simulink model "ActiveLoad_test"  (R2013a)
settings: Solver=ode4  StartTime=0.0  StopTime=10  FixedStep=Ts  RelTol=1e-3
PostLoadFcn:
  | Ts=100e-6; cb_mech_delay=5/60;
InitFcn:
  | Ts=100e-6; cb_mech_delay=5/60;
libraries: breaker_lib x2, powerlib x2, cables_lib x1, transformer_lib x1, alpha_betaActiveLoad_lib x1
settings Model: Creator=ch24070  LastModifiedBy=ed12083

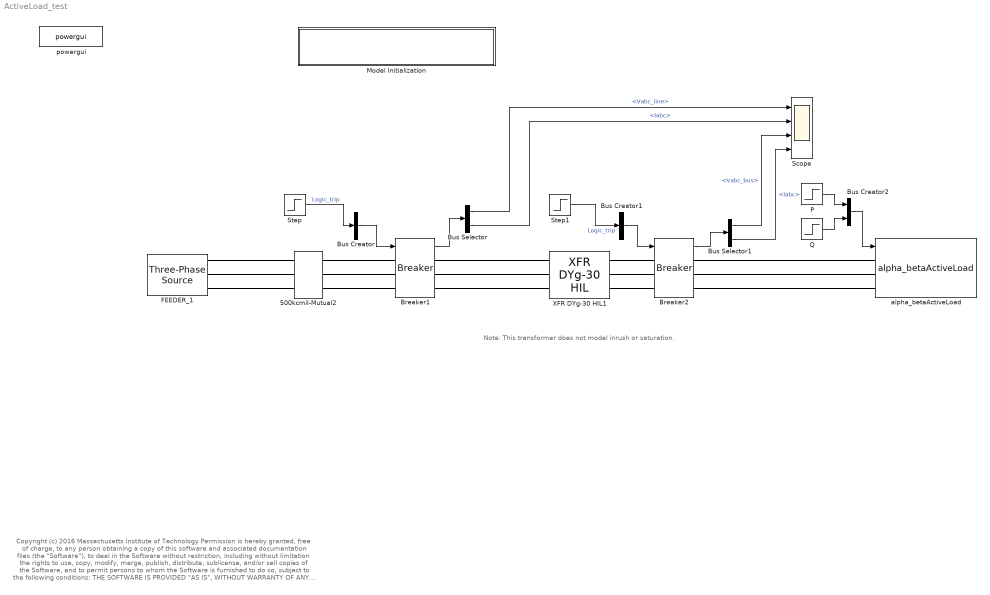
== system ActiveLoad_test ==
  note: Note: This transformer does not model inrush or saturation.
  note: Copyright (c) 2016 Massachusetts Institute of Technology
      | Permission is hereby granted, free of charge, to any person obtaining a copy of this software and associated documentation files (the "Software"), to deal
      | in the Software without restriction, including without limitation the rights to use, copy, modify, merge, publish, distribute, sublicense, and/or sell copies of the
      | Software, and to permit persons to whom the Software is furnished to do so, subject to the following conditions:
      |
      | THE SOFTWARE IS PROVIDED "AS IS", WITHOUT WARRANTY OF ANY KIND, EXPRESS OR IMPLIED, INCLUDING BUT NOT LIMITED TO THE
      | WARRANTIES OF MERCHANTABILITY, FITNESS FOR A PARTICULAR PURPOSE AND NONINFRINGEMENT. IN NO EVENT SHALL THE AUTHORS
      | OR COPYRIGHT HOLDERS BE LIABLE FOR ANY CLAIM, DAMAGES OR OTHER LIABILITY, WHETHER IN AN ACTION OF CONTRACT, TORT OR
      | OTHERWISE, ARISING FROM, OUT OF OR IN CONNECTION WITH THE SOFTWARE OR THE USE OR OTHER DEALINGS IN THE SOFTWARE.
  500kcmil-Mutual2 : cables_lib/500kcmil-Mutual  length=5000  par_sets=1  ratio=3
  Breaker1 : breaker_lib/Breaker  Ts=Ts  mech_delay=cb_mech_delay
  Breaker2 : breaker_lib/Breaker  Ts=Ts  mech_delay=cb_mech_delay
  Bus Creator : BusCreator  Inputs=1
  Bus Creator1 : BusCreator  Inputs=1
  Bus Creator2 : BusCreator  Inputs=2
  Bus Selector : BusSelector  OutputSignals=Vabc_line,Iabc
  Bus Selector1 : BusSelector  OutputSignals=Vabc_bus,Iabc
  FEEDER_1 : powerlib/Electrical Sources/Three-Phase Source  Voltage=13800  PhaseAngle=0  Frequency=60  InternalConnection=Yg  SpecifyImpedance=on  Resistance=0.8929  Inductance=16.58e-3  ShortCircuitLevel=375e6  BaseVoltage=13800  XRratio=7.9  BusType=swing  Pref=0  Qref=0  Qmin=-inf  Qmax=inf
  Model Initialization : Subsystem  AncestorBlock=artemis/Tools /Misc/Model Initialization  mask(Model Functions){InitFcnX=Ts=100e-6; cb_mech_delay=5/60;, prel=off, posl=on, inif=on, strf=off}
      mask prompts: InitFcnX "Initialisation"; prel "Preload Function"; posl "PostLoad Function"; inif "InitFcn"; strf "StartFcn"
      mask init:
      | currentBlock = gcb;
      | root = bdroot(currentBlock);
      | 
      | 
      | if ~strcmp(get_param(root,'BlockDiagramType'),'library')
      |     if prel==1
      |         set_param(root, 'PreLoadFcn', InitFcnX);
      |     else
      |         set_param(root, 'PreLoadFcn', '');
      |     end
      |     if inif==1
      |         set_param(root, 'InitFcn', InitFcnX);
      |     else
      |         set_param(root, 'InitFcn', '');
      |     end
      |     if strf==1
      |         set_param(root, 'StartFcn', InitFcnX);
      |     else
      |         set_param(root, 'StartFcn', '');
      |     end
      |     if posl==1
      |         set_param(root, 'PostLoadFcn', InitFcnX);
      |     else
      |         set_param(root, 'PostLoadFcn', '');
      |     end
      | end
      | 
      | pos = get_param(currentBlock, 'Position');
      | width = pos(3) - pos(1); height = pos(4) - pos(2);
      | txt = [ upper(root) '\n' '- InitFcn. . . . . '  get_param(root, 'InitFcn') ];
      settings: CopyFcn=set_param(gcb,'LinkStatus','inactive')
      mask Display: text(5, height*0.5, txt, 'horizontalAlignment', 'left', 'verticalAlignment', 'middle') ;
  P : Step  Time=5  Before=500  After=0  SampleTime=0
  Q : Step  Time=5  After=500  SampleTime=0
  Scope : Scope  NumInputPorts=4
      settings: YMin=-12500~-150~-400~-4000  YMax=12500~150~400~4000
  Step : Step  SampleTime=0
  Step1 : Step  Time=2  SampleTime=0
  XFR DYg-30 HIL1 : transformer_lib/XFR DYg-30 HIL  Rating=2500  Vp=13800  Vs=480  Z=5.18  XR=2.5
  alpha_betaActiveLoad : alpha_betaActiveLoad_lib/alpha_betaActiveLoad  V=480
  powergui : powerlib/powergui  Priority=2  SimulationMode=Discrete  SolverType=Tustin  SampleTime=Ts  frequency=60  SPID=off  DisableSnubberDevices=off  DisableRonSwitches=off  DisableVfSwitches=off  SwTol=0  Interpol=off  DisplayEquations=off  frequencyindice=0  Pbase=100e6  ErrMax=1e-4  Iterations=50  UnitsV=kV  UnitsW=MW  FunctionMessages=off  echomessages=off  HookPort=off  EnableUseOfTLC=off  x0status=blocks  RestoreLinks=warning  ResistiveCurrentMeasurement=off  Frange=logspace(0,3,50)  Ylog=off  Xlog=off  ShowGrid=off  save=off  variable=ZData  structure=0  ZoomFFT=on  StartTime=0.0  cycles=2  DisplayStyle=off  fundamental=60  FreqAxis=off  MaxFrequency=1000  frequencyindicesteady=1  RmsSteady=1  display=off  Ts=0  methode=off
  wires:
  Breaker1/1 -> Bus Selector/1
  Step/1 -> Bus Creator/1  "Logic_trip"
  Bus Creator/1 -> Breaker1/1
  Step1/1 -> Bus Creator1/1  "Logic_trip"
  Bus Creator1/1 -> Breaker2/1
  Breaker2/1 -> Bus Selector1/1
  Bus Selector/1 -> Scope/1  "<Vabc_line>"
  Bus Selector/2 -> Scope/2  "<Iabc>"
  Bus Selector1/1 -> Scope/3  "<Vabc_bus>"
  Bus Selector1/2 -> Scope/4  "<Iabc>"
  Bus Creator2/1 -> alpha_betaActiveLoad/1
  P/1 -> Bus Creator2/1
  Q/1 -> Bus Creator2/2
  connections:
  XFR DYg-30 HIL1/LConn1 -- Breaker1/RConn1
  XFR DYg-30 HIL1/LConn2 -- Breaker1/RConn2
  XFR DYg-30 HIL1/LConn3 -- Breaker1/RConn3
  500kcmil-Mutual2/LConn2 -- FEEDER_1/RConn2
  500kcmil-Mutual2/LConn1 -- FEEDER_1/RConn1
  500kcmil-Mutual2/LConn3 -- FEEDER_1/RConn3
  500kcmil-Mutual2/RConn1 -- Breaker1/LConn1
  500kcmil-Mutual2/RConn2 -- Breaker1/LConn2
  500kcmil-Mutual2/RConn3 -- Breaker1/LConn3
  XFR DYg-30 HIL1/RConn1 -- Breaker2/LConn1
  XFR DYg-30 HIL1/RConn2 -- Breaker2/LConn2
  XFR DYg-30 HIL1/RConn3 -- Breaker2/LConn3
  Breaker2/RConn2 -- alpha_betaActiveLoad/LConn2
  Breaker2/RConn1 -- alpha_betaActiveLoad/LConn1
  Breaker2/RConn3 -- alpha_betaActiveLoad/LConn3

== system ActiveLoad_test/Model Initialization ==
